simulink model "Comau_robot_sim_IK_3dof"  (R2024b)
settings: Solver=FixedStepAuto  StartTime=0.0  StopTime=inf  FixedStep=Ts  RelTol=1e-3
model workspace (MATLAB code in the model file):
  | %% SMART_5NJ_110_3_0_DataFile
  | %============= RigidTransform =============%
  | 
  | %Initialize the RigidTransform structure array by filling in null values.
  | smiDataRobot.RigidTransform(16).translation = [0.0 0.0 0.0];
  | smiDataRobot.RigidTransform(16).angle = 0.0;
  | smiDataRobot.RigidTransform(16).axis = [0.0 0.0 0.0];
  | smiDataRobot.RigidTransform(16).ID = "";
  | 
  | %Translation Method - Cartesian
  | %Rotation Method - Arbitrary Axis
  | smiDataRobot.RigidTransform(1).translation = [0 331 0];  % mm
  | smiDataRobot.RigidTransform(1).angle = 0;  % rad
  | smiDataRobot.RigidTransform(1).axis = [0 0 0];
  | smiDataRobot.RigidTransform(1).ID = "AssemblyGround[SMART-5 NJ-110-3.0 (3D-STEP).STEP-1:SMART-5 NJ-110-3.0_p02.STEP-1]";
  | 
  | %Translation Method - Cartesian
  | %Rotation Method - Arbitrary Axis
  | smiDataRobot.RigidTransform(2).translation = [-450 2240 0];  % mm
  | smiDataRobot.RigidTransform(2).angle = 0;  % rad
  | smiDataRobot.RigidTransform(2).axis = [0 0 0];
  | smiDataRobot.RigidTransform(2).ID = "AssemblyGround[SMART-5 NJ-110-3.0 (3D-STEP).STEP-1:SMART-5 NJ-110-3.0_p05.STEP-1]";
  | 
  | %Translation Method - Cartesian
  | %Rotation Method - Arbitrary Axis
  | smiDataRobot.RigidTransform(3).translation = [-350 830 294.75];  % mm
  | smiDataRobot.RigidTransform(3).angle = 3.1415926535897931;  % rad
  | smiDataRobot.RigidTransform(3).axis = [1 0 0];
  | smiDataRobot.RigidTransform(3).ID = "AssemblyGround[SMART-5 NJ-110-3.0 (3D-STEP).STEP-1:SMART-5 NJ-110-3.0_CR82350080_SM.STEP-1]";
  | 
  | %Translation Method - Cartesian
  | %Rotation Method - Arbitrary Axis
  | smiDataRobot.RigidTransform(4).translation = [-1842.1799999999998 2240 9.9999999999999998e-13];  % mm
  | smiDataRobot.RigidTransform(4).angle = 0;  % rad
  | smiDataRobot.RigidTransform(4).axis = [0 0 0];
  | smiDataRobot.RigidTransform(4).ID = "AssemblyGround[SMART-5 NJ-110-3.0 (3D-STEP).STEP-1:SMART-5 NJ-110-3.0_p08.STEP-1]";
  | 
  | %Translation Method - Cartesian
  | %Rotation Method - Arbitrary Axis
  | smiDataRobot.RigidTransform(5).translation = [-1917.4300000000001 2240 -4.9999999999999997e-12];  % mm
  | smiDataRobot.RigidTransform(5).angle = 1.5707963267948977;  % rad
  | smiDataRobot.RigidTransform(5).axis = [-1.4999999999999981e-15 -1 -1.4999999999999981e-15];
  | smiDataRobot.RigidTransform(5).ID = "AssemblyGround[SMART-5 NJ-110-3.0 (3D-STEP).STEP-1:SMART-5 NJ-110-3.0_CR82350030_SM.STEP-1]";
  | 
  | %Translation Method - Cartesian
  | %Rotation Method - Arbitrary Axis
  | smiDataRobot.RigidTransform(6).translation = [0 0 0];  % mm
  | smiDataRobot.RigidTransform(6).angle = 0;  % rad
  | smiDataRobot.RigidTransform(6).axis = [0 0 0];
  | smiDataRobot.RigidTransform(6).ID = "AssemblyGround[SMART-5 NJ-110-3.0 (3D-STEP).STEP-1:SMART-5 NJ-110-3.0_p01.STEP-1]";
  | 
  | %Translation Method - Cartesian
  | %Rotation Method - Arbitrary Axis
  | smiDataRobot.RigidTransform(7).translation = [-240.25 2190 169.72568626429799];  % mm
  | smiDataRobot.RigidTransform(7).angle = 2.0943951023931966;  % rad
  | smiDataRobot.RigidTransform(7).axis = [0.57735026918962562 -0.57735026918962606 -0.57735026918962562];
  | smiDataRobot.RigidTransform(7).ID = "AssemblyGround[SMART-5 NJ-110-3.0 (3D-STEP).STEP-1:SMART-5 NJ-110-3.0_CR82350050_SM.STEP-1]";
  | 
  | %Translation Method - Cartesian
  | %Rotation Method - Arbitrary Axis
  | smiDataRobot.RigidTransform(8).translation = [-350 830 135.5];  % mm
  | smiDataRobot.RigidTransform(8).angle = 0;  % rad
  | smiDataRobot.RigidTransform(8).axis = [0 0 0];
  | smiDataRobot.RigidTransform(8).ID = "AssemblyGround[SMART-5 NJ-110-3.0 (3D-STEP).STEP-1:SMART-5 NJ-110-3.0_p03.STEP-1]";
  | 
  | %Translation Method - Cartesian
  | %Rotation Method - Arbitrary Axis
  | smiDataRobot.RigidTransform(9).translation = [-350 830 -350.25];  % mm
  | smiDataRobot.RigidTransform(9).angle = 3.1415926535897913;  % rad
  | smiDataRobot.RigidTransform(9).axis = [-0 -0 -1];
  | smiDataRobot.RigidTransform(9).ID = "AssemblyGround[SMART-5 NJ-110-3.0 (3D-STEP).STEP-1:SMART-5 NJ-110-3.0_CR82350070_SM.STEP-2]";
  | 
  | %Translation Method - Cartesian
  | %Rotation Method - Arbitrary Axis
  | smiDataRobot.RigidTransform(10).translation = [-31.217696610640999 802.11016232075008 -179.5];  % mm
  | smiDataRobot.RigidTransform(10).angle = 0;  % rad
  | smiDataRobot.RigidTransform(10).axis = [0 0 0];
  | smiDataRobot.RigidTransform(10).ID = "AssemblyGround[SMART-5 NJ-110-3.0 (3D-STEP).STEP-1:SMART-5 NJ-110-3.0_p06.STEP-1]";
  | 
  | %Translation Method - Cartesian
  | %Rotation Method - Arbitrary Axis
  | smiDataRobot.RigidTransform(11).translation = [-350 830 -194.5];  % mm
  | smiDataRobot.RigidTransform(11).angle = 0.087266462599717279;  % rad
  | smiDataRobot.RigidTransform(11).axis = [0 -1.1451882774215491e-14 -1];
  | smiDataRobot.RigidTransform(11).ID = "AssemblyGround[SMART-5 NJ-110-3.0 (3D-STEP).STEP-1:SMART-5 NJ-110-3.0_p04.STEP-1]";
  | 
  | %Translation Method - Cartesian
  | %Rotation Method - Arbitrary Axis
  | smiDataRobot.RigidTransform(12).translation = [-2007.179999999981 2240.0000000000132 -6.4999999999999995e-11];  % mm
  | smiDataRobot.RigidTransform(12).angle = 0;  % rad
  | smiDataRobot.RigidTransform(12).axis = [0 0 0];
  | smiDataRobot.RigidTransform(12).ID = "AssemblyGround[SMART-5 NJ-110-3.0 (3D-STEP).STEP-1:SMART-5 NJ-110-3.0_p10.STEP-1]";
  | 
  | %Translation Method - Cartesian
  | %Rotation Method - Arbitrary Axis
  | smiDataRobot.RigidTransform(13).translation = [156.75059808498401 472.5 90.5];  % mm
  | smiDataRobot.RigidTransform(13).angle = 2.7734925708571119;  % rad
  | smiDataRobot.RigidTransform(13).axis = [0.1861567878973851 0.69474659060686583 -0.69474659060686583];
  | smiDataRobot.RigidTransform(13).ID = "AssemblyGround[SMART-5 NJ-110-3.0 (3D-STEP).STEP-1:SMART-5 NJ-110-3.0_CR82350070_SM.STEP-1]";
  | 
  | %Translation Method - Cartesian
  | %Rotation Method - Arbitrary Axis
  | smiDataRobot.RigidTransform(14).translation = [-1967.1799999999998 2239.9999999999964 -2.5000000000000001e-11];  % mm
  | smiDataRobot.RigidTransform(14).angle = 1.5707963267948954;  % rad
  | smiDataRobot.RigidTransform(14).axis = [-4.5000000000000005e-15 1 3.5000000000000001e-15];
  | smiDataRobot.RigidTransform(14).ID = "AssemblyGround[SMART-5 NJ-110-3.0 (3D-STEP).STEP-1:SMART-5 NJ-110-3.0_p09.STEP-1]";
  | 
  | %Translation Method - Cartesian
  | %Rotation Method - Arbitrary Axis
  | smiDataRobot.RigidTransform(15).translation = [-495 2239.9999999999982 -2.5000000000000001e-11];  % mm
  | smiDataRobot.RigidTransform(15).angle = 2.0943951023932024;  % rad
  | smiDataRobot.RigidTransform(15).axis = [-0.57735026918962851 -0.57735026918962118 0.57735026918962751];
  | smiDataRobot.RigidTransform(15).ID = "AssemblyGround[SMART-5 NJ-110-3.0 (3D-STEP).STEP-1:SMART-5 NJ-110-3.0_p07.STEP-1]";
  | 
  | %Translation Method - Cartesian
  | %Rotation Method - Arbitrary Axis
  | smiDataRobot.RigidTransform(16).translation = [0 0 0];  % mm
  | smiDataRobot.RigidTransform(16).angle = 0;  % rad
  | smiDataRobot.RigidTransform(16).axis = [0 0 0];
  | smiDataRobot.RigidTransform(16).ID = "RootGround[SMART-5 NJ-110-3.0 (3D-STEP).STEP-1]";
  | 
  | 
  | %============= Solid =============%
  | %Center of Mass (CoM) %Moments of Inertia (MoI) %Product of Inertia (PoI)
  | 
  | %Initialize the Solid structure array by filling in null values.
  | smiDataRobot.Solid(14).mass = 0.0;
  | smiDataRobot.Solid(14).CoM = [0.0 0.0 0.0];
  | smiDataRobot.Solid(14).MoI = [0.0 0.0 0.0];
  | smiDataRobot.Solid(14).PoI = [0.0 0.0 0.0];
  | smiDataRobot.Solid(14).color = [0.0 0.0 0.0];
  | smiDataRobot.Solid(14).opacity = 0.0;
  | smiDataRobot.Solid(14).ID = "";
  | 
  | %Inertia Type - Custom
  | %Visual Properties - Simple
  | smiDataRobot.Solid(1).mass = 52.706031176315982;  % kg
  | smiDataRobot.Solid(1).CoM = [-242.66897813542667 296.14549865714821 12.560965025190244];  % mm
  | smiDataRobot.Solid(1).MoI = [4136639.3686790983 3647453.6565928138 4173251.5664203875];  % kg*mm^2
  | smiDataRobot.Solid(1).PoI = [21269.015167562859 -54887.133975236575 1321088.2058438642];  % kg*mm^2
  | smiDataRobot.Solid(1).color = [0.203 0.210 0.239];
  | smiDataRobot.Solid(1).opacity = 1;
  | smiDataRobot.Solid(1).ID = "SMART-5 NJ-110-3.0_p02.STEP*:*Default";
  | 
  | %Inertia Type - Custom
  | %Visual Properties - Simple
  | smiDataRobot.Solid(2).mass = 25.314195721014904;  % kg
  | smiDataRobot.Solid(2).CoM = [81.922886858874577 -33.833989402443976 14.448782406787638];  % mm
  | smiDataRobot.Solid(2).MoI = [783008.26269064494 548584.67016851983 525604.1322728931];  % kg*mm^2
  | smiDataRobot.Solid(2).PoI = [-112599.38170428496 21299.174138007162 72588.874515329284];  % kg*mm^2
  | smiDataRobot.Solid(2).color = [0.792156862745098 0.81960784313725488 0.93333333333333335];
  | smiDataRobot.Solid(2).opacity = 1;
  | smiDataRobot.Solid(2).ID = "SMART-5 NJ-110-3.0_p05.STEP*:*Default";
  | 
  | %Inertia Type - Custom
  | %Visual Properties - Simple
  | smiDataRobot.Solid(3).mass = 9.4493198216073964;  % kg
  | smiDataRobot.Solid(3).CoM = [0.00035605587580101627 0.59254727846081734 -131.34248514352112];  % mm
  | smiDataRobot.Solid(3).MoI = [96683.905101085853 96090.527287838268 47612.014811029614];  % kg*mm^2
  | smiDataRobot.Solid(3).PoI = [678.15178926669853 -1.9373731491872181 -0.37884372181229253];  % kg*mm^2
  | smiDataRobot.Solid(3).color = [0.792156862745098 0.81960784313725488 0.93333333333333335];
  | smiDataRobot.Solid(3).opacity = 1;
  | smiDataRobot.Solid(3).ID = "SMART-5 NJ-110-3.0_CR82350080_SM.STEP*:*Default";
  | 
  | %Inertia Type - Custom
  | %Visual Properties - Simple
  | smiDataRobot.Solid(4).mass = 27.907822986627043;  % kg
  | smiDataRobot.Solid(4).CoM = [176.91381036358237 3.8341896469272663 1.9754510358205102];  % mm
  | smiDataRobot.Solid(4).MoI = [482005.2410957645 820993.89522460627 552912.66986302414];  % kg*mm^2
  | smiDataRobot.Solid(4).PoI = [-5805.283149630598 -66627.605911827952 -6375.7492384737961];  % kg*mm^2
  | smiDataRobot.Solid(4).color = [0.792156862745098 0.81960784313725488 0.93333333333333335];
  | smiDataRobot.Solid(4).opacity = 1;
  | smiDataRobot.Solid(4).ID = "SMART-5 NJ-110-3.0_p08.STEP*:*Default";
  | 
  | %Inertia Type - Custom
  | %Visual Properties - Simple
  | smiDataRobot.Solid(5).mass = 1.8204370609575367;  % kg
  | smiDataRobot.Solid(5).CoM = [0.0011781120658499607 1.8532136422554566 -83.079832406507592];  % mm
  | smiDataRobot.Solid(5).MoI = [7475.3672830480818 7269.0527134527229 2858.8228291073215];  % kg*mm^2
  | smiDataRobot.Solid(5).PoI = [189.23833790092377 0.076539858692730889 -0.14274057644209939];  % kg*mm^2
  | smiDataRobot.Solid(5).color = [0.792156862745098 0.81960784313725488 0.93333333333333335];
  | smiDataRobot.Solid(5).opacity = 1;
  | smiDataRobot.Solid(5).ID = "SMART-5 NJ-110-3.0_CR82350030_SM.STEP*:*Default";
  | 
  | %Inertia Type - Custom
  | %Visual Properties - Simple
  | smiDataRobot.Solid(6).mass = 98.712536679746705;  % kg
  | smiDataRobot.Solid(6).CoM = [36.183943831325131 132.25114554111747 -0.030525648643372944];  % mm
  | smiDataRobot.Solid(6).MoI = [3268478.8711421788 6102276.4254572866 4269111.0143532446];  % kg*mm^2
  | smiDataRobot.Solid(6).PoI = [-35.583053939592197 631.47068636807955 -2524.4017230519235];  % kg*mm^2
  | smiDataRobot.Solid(6).color = [0.792156862745098 0.81960784313725488 0.93333333333333335];
  | smiDataRobot.Solid(6).opacity = 1;
  | smiDataRobot.Solid(6).ID = "SMART-5 NJ-110-3.0_p01.STEP*:*Default";
  | 
  | %Inertia Type - Custom
  | %Visual Properties - Simple
  | smiDataRobot.Solid(7).mass = 3.5666359355844257;  % kg
  | smiDataRobot.Solid(7).CoM = [1.2461000205248818 -0.0010192432622059655 -85.200466358919499];  % mm
  | smiDataRobot.Solid(7).MoI = [17145.157040564802 17509.336534066519 10295.619245635809];  % kg*mm^2
  | smiDataRobot.Solid(7).PoI = [-0.163954126982988 300.11359564551077 0.32104894325969818];  % kg*mm^2
  | smiDataRobot.Solid(7).color = [0.6392157 0.0 0.0];
  | smiDataRobot.Solid(7).opacity = 1;
  | smiDataRobot.Solid(7).ID = "SMART-5 NJ-110-3.0_CR82350050_SM.STEP*:*Default";
  | 
  | %Inertia Type - Custom
  | %Visual Properties - Simple
  | smiDataRobot.Solid(8).mass = 22.854890403146104;  % kg
  | smiDataRobot.Solid(8).CoM = [-23.928506665749911 523.99566525340538 -159.70044895169784];  % mm
  | smiDataRobot.Solid(8).MoI = [3177590.9155515293 341455.30737882649 3069690.399421786];  % kg*mm^2
  | smiDataRobot.Solid(8).PoI = [51188.540610659591 -6971.0396180961588 7197.3923801430437];  % kg*mm^2
  | smiDataRobot.Solid(8).color = [0.64 0.0 0.0];
  | smiDataRobot.Solid(8).opacity = 1;
  | smiDataRobot.Solid(8).ID = "SMART-5 NJ-110-3.0_p03.STEP*:*Default";
  | 
  | %Inertia Type - Custom
  | %Visual Properties - Simple
  | smiDataRobot.Solid(9).mass = 8.5814594224327365;  % kg
  | smiDataRobot.Solid(9).CoM = [0.00039190881468678792 0.65247306493897117 -117.33220651590989];  % mm
  | smiDataRobot.Solid(9).MoI = [76220.255867257161 75627.213475154422 43301.239657847611];  % kg*mm^2
  | smiDataRobot.Solid(9).PoI = [598.99194041261785 -1.5272912821901943 -0.37849880267797315];  % kg*mm^2
  | smiDataRobot.Solid(9).color = [0.792156862745098 0.81960784313725488 0.93333333333333335];
  | smiDataRobot.Solid(9).opacity = 1;
  | smiDataRobot.Solid(9).ID = "SMART-5 NJ-110-3.0_CR82350070_SM.STEP*:*Default";
  | 
  | %Inertia Type - Custom
  | %Visual Properties - Simple
  | smiDataRobot.Solid(10).mass = 7.5792666918117497;  % kg
  | smiDataRobot.Solid(10).CoM = [65.147048462687252 508.83792056545542 14.747257945702893];  % mm
  | smiDataRobot.Solid(10).MoI = [667373.64067244437 18083.172326137388 678945.36689657171];  % kg*mm^2
  | smiDataRobot.Solid(10).PoI = [-225.7042116055666 46.998810275833364 17500.803228922214];  % kg*mm^2
  | smiDataRobot.Solid(10).color = [0.792156862745098 0.81960784313725488 0.93333333333333335];
  | smiDataRobot.Solid(10).opacity = 1;
  | smiDataRobot.Solid(10).ID = "SMART-5 NJ-110-3.0_p06.STEP*:*Default";
  | 
  | %Inertia Type - Custom
  | %Visual Properties - Simple
  | smiDataRobot.Solid(11).mass = 4.3287759696132397;  % kg
  | smiDataRobot.Solid(11).CoM = [163.57070996069299 -9.8617817182830834 27.536485713357724];  % mm
  | smiDataRobot.Solid(11).MoI = [15456.864188549995 65374.86371961276 72810.661297813465];  % kg*mm^2
  | smiDataRobot.Solid(11).PoI = [-165.91415506329329 512.48565629209236 3817.7544015007338];  % kg*mm^2
  | smiDataRobot.Solid(11).color = [0.792156862745098 0.81960784313725488 0.93333333333333335];
  | smiDataRobot.Solid(11).opacity = 1;
  | smiDataRobot.Solid(11).ID = "SMART-5 NJ-110-3.0_p04.STEP*:*Default";
  | 
  | %Inertia Type - Custom
  | %Visual Properties - Simple
  | smiDataRobot.Solid(12).mass = 0.47985825240457192;  % kg
  | smiDataRobot.Solid(12).CoM = [-27.34791626851143 -1.6026209534547153 -5.1001180974803206e-05];  % mm
  | smiDataRobot.Solid(12).MoI = [1618.4776017805987 894.29456427734294 837.21364973354628];  % kg*mm^2
  | smiDataRobot.Solid(12).PoI = [-7.7780608542633322e-06 0.00054638186946613686 4.4070273941284572];  % kg*mm^2
  | smiDataRobot.Solid(12).color = [0.792156862745098 0.81960784313725488 0.93333333333333335];
  | smiDataRobot.Solid(12).opacity = 1;
  | smiDataRobot.Solid(12).ID = "SMART-5 NJ-110-3.0_p10.STEP*:*Default";
  | 
  | %Inertia Type - Custom
  | %Visual Properties - Simple
  | smiDataRobot.Solid(13).mass = 2.1916043056807371;  % kg
  | smiDataRobot.Solid(13).CoM = [-0.46659407311739648 -0.96652135243620041 26.711273550845025];  % mm
  | smiDataRobot.Solid(13).MoI = [11436.827713254688 13423.173203473376 8596.8063115297427];  % kg*mm^2
  | smiDataRobot.Solid(13).PoI = [153.22479160131755 -298.20565802941911 -10.064478096809076];  % kg*mm^2
  | smiDataRobot.Solid(13).color = [0.792156862745098 0.81960784313725488 0.93333333333333335];
  | smiDataRobot.Solid(13).opacity = 1;
  | smiDataRobot.Solid(13).ID = "SMART-5 NJ-110-3.0_p09.STEP*:*Default";
  | 
  | %Inertia Type - Custom
  | %Visual Properties - Simple
  | smiDataRobot.Solid(14).mass = 18.744700041112438;  % kg
  | smiDataRobot.Solid(14).CoM = [-0.005958152306662661 -0.089401100201608463 460.33855874646821];  % mm
  | smiDataRobot.Solid(14).MoI = [1632832.4693022415 1632553.6239231301 67074.935683703909];  % kg*mm^2
  | smiDataRobot.Solid(14).PoI = [-835.38260715793831 53.677126594132538 -8.4899136334609864];  % kg*mm^2
  | smiDataRobot.Solid(14).color = [0.792156862745098 0.81960784313725488 0.93333333333333335];
  | smiDataRobot.Solid(14).opacity = 1;
  | smiDataRobot.Solid(14).ID = "SMART-5 NJ-110-3.0_p07.STEP*:*Default";
values from neighbouring files (symbols this model uses):
  M = [1 0 0 L1+L5+L6+L7 ... (first row only)    [Comau_robot_3dof_parameters.m]
  SList = [omega_mat; v_mat]    [Comau_robot_3dof_parameters.m]
  thetaList0 = [0 0 0 0 0]    [Comau_robot_3dof_parameters.m]
undefined symbols (not defined in the file or in its folder): L2, L3, L4, smiDataRobot, X, Y, Z
libraries: sm_lib x85, nesl_utility x31, slrealtimeutilitieslib x1, slrealtimeiplib x1, aerolibanimutils x1
(part 1 of 5)
settings Model: Creator=jojoa  LastModifiedBy=Thoma

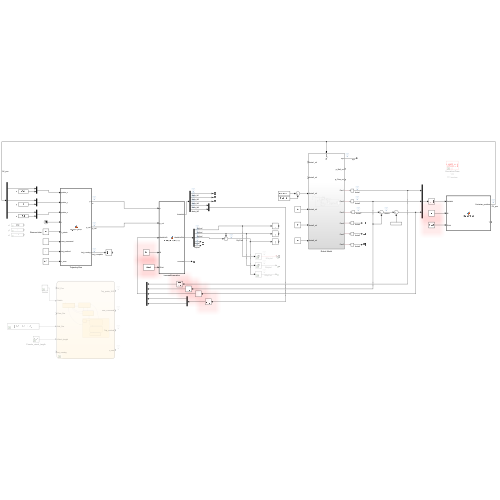
[thumbnail: Simulink's stored preview of the top-level diagram]
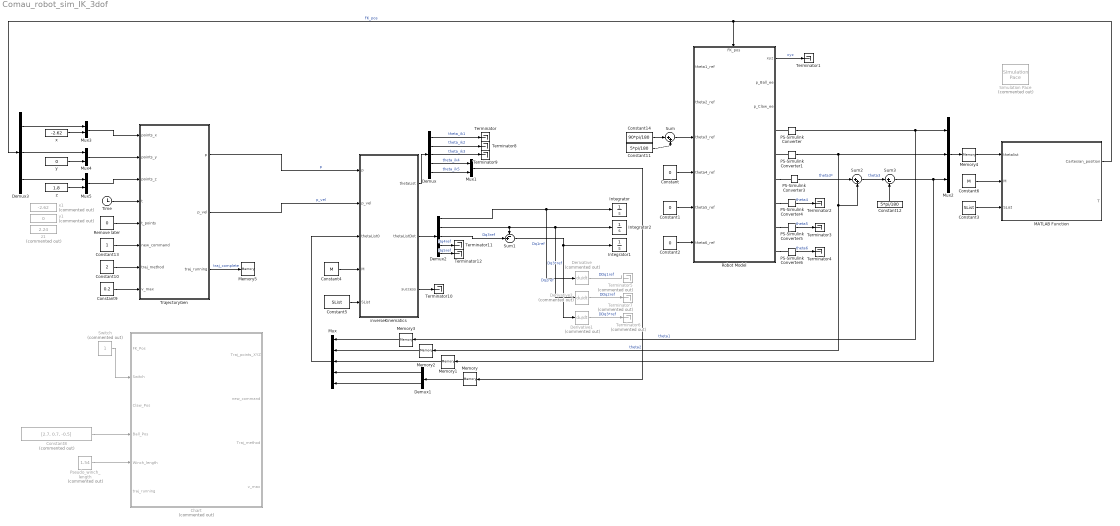
== system Comau_robot_sim_IK_3dof ==
  Chart : Stateflow chart  Commented=on  TreatAsAtomicUnit=on
      settings: PortSchema="{\"entries\":[{\"content\":{\"sides\":[{\"content\":{\"connectorIds\":[\"In2\",\"In1\",\"In3\",\"In4\",\"In5\",\"In6\"]},\"type\":\"ConnectorPlacement.EquallySpacedRectSide\",\"uuid\":\"172fb156-0aeb-45d6-ae82-af15bd6c897e\"},{\"content\":{\"connectorIds\":[\"Out1\",\"Out2\",\"Out3\",\"Out4\"],\"side\":\"RIGHT\"},\"type\":\"ConnectorPlacement.EquallySpacedRectSide\",\"uuid\":\"236a4085-9b1e-46f1-9589-a1369625993a\"},{\"content\":{\"side\":\"TOP\"},\"type\":\"ConnectorPlacement.EquallySpacedRectSide\",\"uuid\":\"81d2e992-6e31-4ebe-a88a-0042095fc779\"}]},\"type\":\"ConnectorPlacement.EquallySpacedConnector\",\"uuid\":\"b030cd03-88b5-40ca-9a91-4cb72ee04091\"}],\"packageUris\":[\"http://schema.mathworks.com/mf0/Connector/R2020b\"],\"version\":\"1.0\"}"
  Constant : Constant  Value=0
  Constant1 : Constant  Value=0
  Constant10 : Constant  Value=2
  Constant11 : Constant  Value=5*pi/180
  Constant12 : Constant  Value=5*pi/180
  Constant13 : Constant
  Constant14 : Constant  Value=90*pi/180
  Constant2 : Constant  Value=0
  Constant3 : Constant  Value=SList
  Constant4 : Constant  Value=M
  Constant5 : Constant  Value=SList
  Constant6 : Constant  Value=M
  Constant8 : Constant  Commented=on  Value=[2.7, 0.7, -0.5]
  Constant9 : Constant  Value=0.2
  Demux : Demux  Outputs=5
  Demux1 : Demux  Outputs=2
  Demux2 : Demux  Outputs=5
  Demux3 : Demux  Outputs=3
  Derivative : Derivative  Commented=on
  Derivative1 : Derivative  Commented=on
  Derivative2 : Derivative  Commented=on
  Integrator : Integrator
  Integrator1 : Integrator
  Integrator2 : Integrator
  MATLAB Function : MATLAB Function  TreatAsAtomicUnit=on
  Memory : Memory  InitialCondition=[thetaList0(4), thetaList0(5)]
  Memory1 : Memory  InitialCondition=thetaList0(3)
  Memory2 : Memory  InitialCondition=thetaList0(2)
  Memory3 : Memory  InitialCondition=thetaList0(1)
  Memory4 : Memory
  Memory5 : Memory
  Mux : Mux  Inputs=5
  Mux{1,3..5} (4 alike) : Mux  Inputs=2
  Mux2 : Mux  Inputs=3
  PS-Simulink Converter{,1,3..6} (6 alike) : nesl_utility/PS-Simulink Converter  PhysicalDomain=network_engine_domain  SubClassName=ps_output  LeftPortType=input  RightPortType=output  PseudoPeriodic=off  Frequencies=[]  VectorFormat=inherit  Unit=inherit  AffineConversion=off
  Pseudo_winch_length : Constant  Commented=on  Value=1.54
  Remove later : Constant  Value=0
  Robot Model : Subsystem
      settings: PortSchema="{\"entries\":[{\"content\":{\"sides\":[{\"content\":{\"connectorIds\":[\"In1\",\"In2\",\"In3\",\"In4\",\"In5\",\"In6\"]},\"type\":\"ConnectorPlacement.EquallySpacedRectSide\",\"uuid\":\"6aa2e516-c804-4755-b4dc-c78d50aa59d9\"},{\"content\":{\"connectorIds\":[\"Out1\",\"Out2\",\"Out3\",\"RConn1\",\"RConn2\",\"RConn3\",\"RConn4\",\"RConn5\",\"RConn6\"],\"side\":\"RIGHT\"},\"type\":\"ConnectorPlacement.EquallySpacedRectSide\",\"uuid\":\"639c1142-9616-4d5f-b210-c20b0bbda392\"},{\"content\":{\"connectorIds\":[\"In7\"],\"side\":\"TOP\"},\"type\":\"ConnectorPlacement.EquallySpacedRectSide\",\"uuid\":\"5b61a740-c71f-4d58-86f2-86cfe83aa5ec\"}]},\"type\":\"ConnectorPlacement.EquallySpacedConnector\",\"uuid\":\"c7a9e42c-08d7-4193-b201-c243b42c995e\"}],\"packageUris\":[\"http://schema.mathworks.com/mf0/Connector/R2020b\"],\"version\":\"1.0\"}"
  Simulation Pace : aerolibanimutils/Simulation Pace  Commented=on  SimulationPace=1  SleepMode=Auto  OutputPaceError=off  SampleTime=0.001
  Sum : Sum  Inputs=|++
  Sum1 : Sum  Inputs=-+|
  Sum2 : Sum  Inputs=|++
  Sum3 : Sum  Inputs=|+-
  Switch : Constant  Commented=on
  Terminator{,1..4,8..12} (10 alike) : Terminator
  Terminator5 : Terminator  Commented=on
  Terminator6 : Terminator  Commented=on
  Terminator7 : Terminator  Commented=on
  Time : Clock
  TrajectoryGen : MATLAB Function  TreatAsAtomicUnit=on
  inverseKinematics : MATLAB Function  TreatAsAtomicUnit=on
  x : Constant  Value=-2.62
  x1 : Constant  Commented=on  Value=-2.62
  y : Constant  Value=0
  y1 : Constant  Commented=on  Value=0
  z : Constant  Value=1.8
  z1 : Constant  Commented=on  Value=2.24
  wires:
  PS-Simulink Converter/1 -> Memory3/1, Mux2/1  "theta1"
  Robot Model/1(xyz) -> Terminator1/1  "xyz"
  Mux/1 -> inverseKinematics/3(thetaList0)
  Memory3/1 -> Mux/1
  Constant5/1 -> inverseKinematics/5(SList)
  Memory2/1 -> Mux/2
  inverseKinematics/1(thetaList) -> Demux/1
  Constant4/1 -> inverseKinematics/4(M)
  inverseKinematics/2(thetaListDot) -> Demux2/1
  Demux2/1 -> Derivative/1, Integrator/1  "Dq1ref"
  Demux2/4 -> Terminator11/1  "Dq4ref"
  Demux2/5 -> Terminator12/1  "Dq5ref"
  Memory/1 -> Demux1/1
  Demux1/1 -> Mux/4
  Demux1/2 -> Mux/5
  Demux/4 -> Mux1/1  "theta_ik4"
  Demux/5 -> Mux1/2  "theta_ik5"
  Constant/1 -> Robot Model/4(theta4_ref)
  Constant1/1 -> Robot Model/5(theta5_ref)
  Constant2/1 -> Robot Model/6(theta6_ref)
  Demux2/2 -> Sum1/1, Derivative2/1, Integrator2/1  "Dq2ref"
  Mux2/1 -> Memory4/1
  Constant6/1 -> MATLAB Function/2(M)
  Constant3/1 -> MATLAB Function/3(SList)
  PS-Simulink Converter4/1 -> Terminator2/1  "theta4"
  PS-Simulink Converter5/1 -> Terminator3/1  "theta5"
  PS-Simulink Converter6/1 -> Terminator4/1  "theta6"
  Time/1 -> TrajectoryGen/4(t)
  Mux1/1 -> Memory/1
  PS-Simulink Converter1/1 -> Sum2/2, Memory2/1, Mux2/2  "theta2"
  Memory1/1 -> Mux/3
  PS-Simulink Converter3/1 -> Sum2/1  "theta3*"
  Sum1/1 -> Derivative1/1, Integrator1/1  "Dq3*ref"
  Demux2/3 -> Sum1/2  "Dq3ref"
  Derivative/1 -> ?  "DDq1ref"
  Derivative1/1 -> Terminator6/1  "DDq3*ref"
  Derivative2/1 -> Terminator7/1  "DDq2ref"
  Constant11/1 -> Sum/2
  Sum2/1 -> Sum3/1  "theta3"
  Constant12/1 -> Sum3/2
  Sum3/1 -> Memory1/1, Mux2/3
  TrajectoryGen/1(p) -> inverseKinematics/1(p)  "p"
  TrajectoryGen/2(p_vel) -> inverseKinematics/2(p_vel)  "p_vel"
  MATLAB Function/1(Cartesian_position) -> Demux3/1, Robot Model/7(FK_pos)  "FK_pos"
  Memory4/1 -> MATLAB Function/1(thetalist)
  Demux/1 -> Terminator/1  "theta_ik1"
  Demux/2 -> Terminator8/1  "theta_ik2"
  Demux/3 -> Terminator9/1  "theta_ik3"
  inverseKinematics/3(success) -> Terminator10/1
  x/1 -> Mux3/2
  Demux3/1 -> Mux3/1
  Demux3/2 -> Mux4/1
  y/1 -> Mux4/2
  Demux3/3 -> Mux5/1
  z/1 -> Mux5/2
  Remove later/1 -> TrajectoryGen/5(t_points)
  Switch/1 -> Chart/1(Switch)
  Sum/1 -> Robot Model/3(theta3_ref)
  TrajectoryGen/3(traj_running) -> Memory5/1  "traj_complete"
  Pseudo_winch_length/1 -> Chart/5(Winch_length)
  Constant8/1 -> Chart/4(Ball_Pos)
  Mux3/1 -> TrajectoryGen/1(points_x)
  Mux4/1 -> TrajectoryGen/2(points_y)
  Mux5/1 -> TrajectoryGen/3(points_z)
  Constant9/1 -> TrajectoryGen/8(v_max)
  Constant10/1 -> TrajectoryGen/7(traj_method)
  Constant13/1 -> TrajectoryGen/6(new_command)
  Constant14/1 -> Sum/1
  connections:
  Robot Model/RConn4 -- PS-Simulink Converter4/LConn1
  PS-Simulink Converter/LConn1 -- Robot Model/RConn1
  Robot Model/RConn5 -- PS-Simulink Converter5/LConn1
  Robot Model/RConn3 -- PS-Simulink Converter3/LConn1
  PS-Simulink Converter1/LConn1 -- Robot Model/RConn2
  Robot Model/RConn6 -- PS-Simulink Converter6/LConn1
